simulink model "impedance_target"  (R2021b)
settings: Solver=ode1  StartTime=0.0  StopTime=inf  FixedStep=2e-4  RelTol=1e-3  EnableMultiTasking=on
InitFcn:
  | current_gain = 0.05;
libraries: spsSecondOrderFilterLib x4, speedgoatlib_IO102 x3, slrealtimeutilitieslib x1, slrealtimeiplib x1
settings Model: sg_rtwmakecfg_data=_sglibc_  SimulationMode=external  Creator=tcraddoc  LastModifiedBy=wasynczu
settings SolverCC: ConcurrentTasks=on  AlgebraicLoopSolver=TrustRegion  PositivePriorityOrder=on
settings DataIOCC: SaveFormat=StructureWithTime  ReturnWorkspaceOutputs=off
settings OptimizationCC: BlockReduction=off  OptimizeBlockIOStorage=off  BufferReuse=off  GlobalBufferReuse=off  ExpressionFolding=off  LocalBlockOutputs=off  OptimizeDataStoreBuffers=off  BusAssignmentInplaceUpdate=off
settings DebuggingCC: TasksWithSamePriorityMsg=none  SFMachineParentedDataDiag=warning  ArithmeticOperatorsInVariantConditions=warning
settings HardwareCC: ProdBitPerLong=64  ProdLongLongMode=on  ProdHWDeviceType=Intel->x86-64 (Linux 64)
settings SFSimCC: SimUseLocalCustomCode=off  CustomCodeUndefinedFunction=UseInterfaceOnly
settings RTWCC: Description=Simulink Real-Time  SystemTargetFile=slrealtime.tlc  TemplateMakefile=slrealtime_default_tmf  RTWUseLocalCustomCode=off  Toolchain=Simulink Real-Time Toolchain  BuildConfiguration=Faster Runs  CodeExecutionProfiling=on  TargetLang=C++
settings CodeAppCC: StateflowObjectComments=on
settings SimscapeCC: SimscapeNormalizeSystem=off

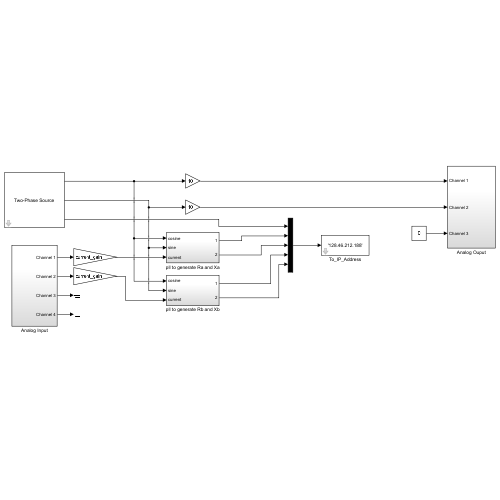
[thumbnail: Simulink's stored preview of the top-level diagram]
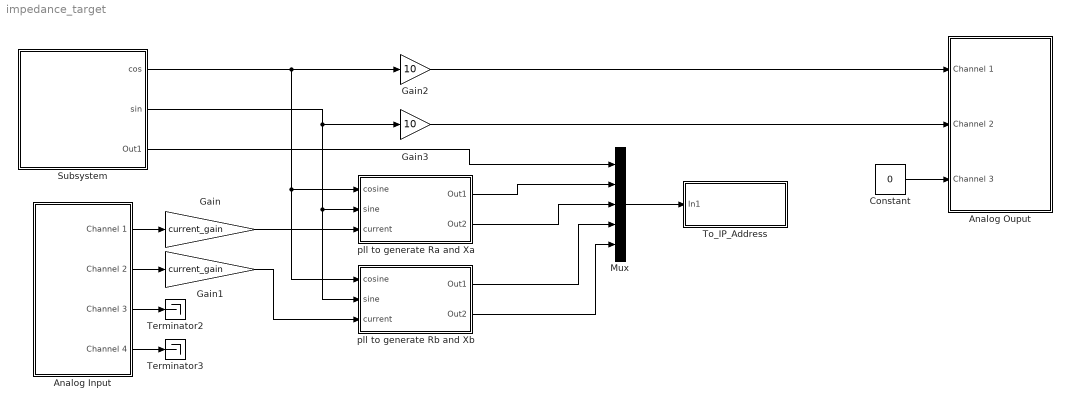
== system impedance_target ==
  Analog Input : Subsystem
  Analog Ouput : Subsystem
  Constant : Constant  Value=0
  Gain : Gain  Gain=current_gain
  Gain1 : Gain  Gain=current_gain
  Gain2 : Gain  Gain=10
  Gain3 : Gain  Gain=10
  Mux : Mux  Inputs=5
  Subsystem : Subsystem  mask{freq=10}
      mask prompts: freq "Frequency (Hz)"
      mask Display: disp('Two-Phase Source')
  Terminator2 : Terminator
  Terminator3 : Terminator
  To_IP_Address : Subsystem  mask{toAddress='128.46.212.188'}
      mask prompts: toAddress "To IP address"
      mask Display: disp(get_param(gcb,'toAddress'))
  pll to generate Ra and Xa : Subsystem
  pll to generate Rb and Xb : Subsystem
  wires:
  Subsystem/1(cos) -> pll to generate Rb and Xb/1(cosine), pll to generate Ra and Xa/1(cosine), Gain2/1
  Constant/1 -> Analog Ouput/3(Channel 3)
  Analog Input/1(Channel 1) -> Gain/1
  Analog Input/2(Channel 2) -> Gain1/1
  Analog Input/4(Channel 4) -> Terminator3/1
  Analog Input/3(Channel 3) -> Terminator2/1
  Subsystem/2(sin) -> pll to generate Rb and Xb/2(sine), pll to generate Ra and Xa/2(sine), Gain3/1
  Gain/1 -> pll to generate Ra and Xa/3(current)
  Gain1/1 -> pll to generate Rb and Xb/3(current)
  Gain2/1 -> Analog Ouput/1(Channel 1)
  Gain3/1 -> Analog Ouput/2(Channel 2)
  Subsystem/3(Out1) -> Mux/1
  pll to generate Ra and Xa/1(Out1) -> Mux/2
  pll to generate Ra and Xa/2(Out2) -> Mux/3
  pll to generate Rb and Xb/1(Out1) -> Mux/4
  pll to generate Rb and Xb/2(Out2) -> Mux/5
  Mux/1 -> To_IP_Address/1(In1)

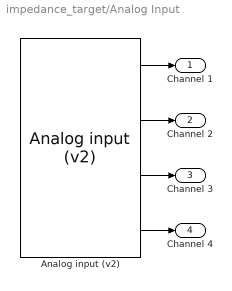
== system impedance_target/Analog Input ==
  "Analog input (v2) " : speedgoatlib_IO102/Analog input (v2)   id=1  channels=[1 2 3 4]  range=1  high_voltage=off  adCoupling=2  ts=2e-4  pciSlot=-1
      settings: SourceProductName=Simulink Real-Time: Speedgoat I/O Blockset
  Channel 1 : Outport
  Channel 2 : Outport  Port=2
  Channel 3 : Outport  Port=3
  Channel 4 : Outport  Port=4
  wires:
  "Analog input (v2) "/4 -> Channel 4/1
  "Analog input (v2) "/2 -> Channel 2/1
  "Analog input (v2) "/1 -> Channel 1/1
  "Analog input (v2) "/3 -> Channel 3/1

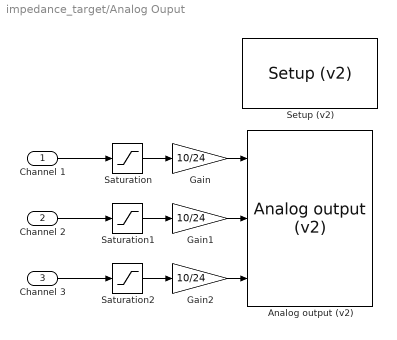
== system impedance_target/Analog Ouput ==
  Channel 1 : Inport
  Channel 2 : Inport  Port=2
  Channel 3 : Inport  Port=3
  "Analog output (v2) " : speedgoatlib_IO102/Analog output (v2)   id=1  channels=[1 2 3]  range=1  ts=2e-4  pciSlot=-1
      settings: SourceProductName=Simulink Real-Time: Speedgoat I/O Blockset
  Gain : Gain  Gain=10/24
  Gain1 : Gain  Gain=10/24
  Gain2 : Gain  Gain=10/24
  Saturation : Saturate  UpperLimit=24  LowerLimit=-24
  Saturation1 : Saturate  UpperLimit=24  LowerLimit=-24
  Saturation2 : Saturate  UpperLimit=24  LowerLimit=-24
  "Setup (v2) " : speedgoatlib_IO102/Setup (v2)   id=1  range=+-10V  cal=off  pciSlot=-1  adCoupling=Single-ended  adChannelMode=Multiple-channel (enter number of channels below)  adChannel=4  daChannel=[1,2,3]  daInitValue=[0]  daReset=[1]  DioDirectionLo=Input  DioDirectionHi=Output  doChannel=[9]  doInitValue=[0]  doReset=[1]  diChannel=[1]
      settings: SourceProductName=Simulink Real-Time: Speedgoat I/O Blockset
  wires:
  Saturation/1 -> Gain/1
  Saturation1/1 -> Gain1/1
  Saturation2/1 -> Gain2/1
  Gain1/1 -> "Analog output (v2) "/2
  Gain/1 -> "Analog output (v2) "/1
  Gain2/1 -> "Analog output (v2) "/3
  Channel 2/1 -> Saturation1/1
  Channel 3/1 -> Saturation2/1
  Channel 1/1 -> Saturation/1

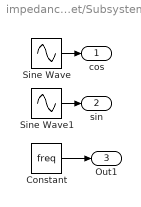
== system impedance_target/Subsystem ==
  Constant : Constant  Value=freq
  Sine Wave : Sin  Frequency=2*pi*freq  Phase=pi/2  SampleTime=0
  Sine Wave1 : Sin  Frequency=2*pi*freq  SampleTime=0
  cos : Outport  VectorParamsAs1DForOutWhenUnconnected=off
  sin : Outport  Port=2  VectorParamsAs1DForOutWhenUnconnected=off
  Out1 : Outport  Port=3
  wires:
  Sine Wave1/1 -> sin/1
  Sine Wave/1 -> cos/1
  Constant/1 -> Out1/1

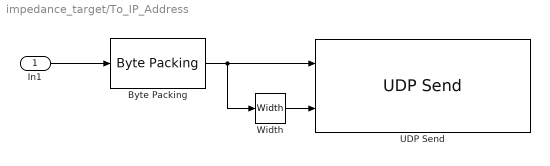
== system impedance_target/To_IP_Address ==
  In1 : Inport
  Byte Packing : slrealtimeutilitieslib/Byte Packing  MaskPackedDataType=uint8  MaskUnpackedDataTypes={['double']}  MaskAlignment=1
  UDP Send : slrealtimeiplib/UDP Send  useHostTargetConn=on  toAddress=toAddress  toPort=34  sampleTime=-1
      settings: SourceProductBaseCode=XP
  Width : Width
  wires:
  In1/1 -> Byte Packing/1
  Byte Packing/1 -> Width/1, UDP Send/1
  Width/1 -> UDP Send/2

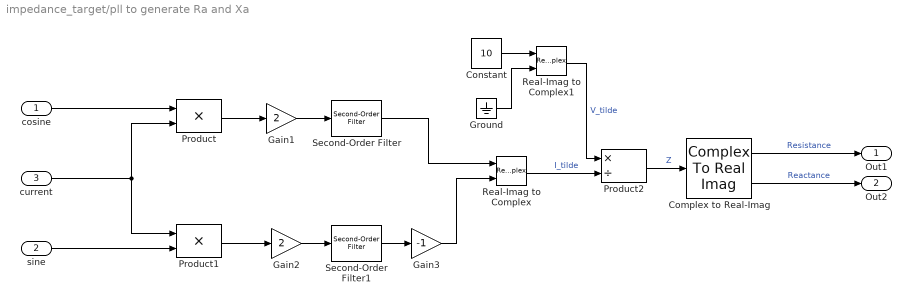
== system impedance_target/pll to generate Ra and Xa ==
  cosine : Inport
  sine : Inport  Port=2
  current : Inport  Port=3
  Complex to Real-Imag : ComplexToRealImag
  Constant : Constant  Value=10
  Gain1 : Gain  Gain=2  SaturateOnIntegerOverflow=on  OutDataTypeStr=Inherit: Same as input  ParamDataTypeStr=Inherit: Same as input
  Gain2 : Gain  Gain=2  SaturateOnIntegerOverflow=on  OutDataTypeStr=Inherit: Same as input  ParamDataTypeStr=Inherit: Same as input
  Gain3 : Gain  Gain=-1  SaturateOnIntegerOverflow=on  OutDataTypeStr=Inherit: Same as input  ParamDataTypeStr=Inherit: Same as input
  Ground : Ground
  Product : Product  InputSameDT=on  SaturateOnIntegerOverflow=on  OutDataTypeStr=Inherit: Same as first input
  Product1 : Product  InputSameDT=on  SaturateOnIntegerOverflow=on  OutDataTypeStr=Inherit: Same as first input
  Product2 : Product  Inputs=*/  InputSameDT=on  SaturateOnIntegerOverflow=on  OutDataTypeStr=Inherit: Same as first input
  Real-Imag to Complex : RealImagToComplex
  Real-Imag to Complex1 : RealImagToComplex
  Second-Order Filter : spsSecondOrderFilterLib/Second-Order Filter  FilterType=Lowpass  Fo=0.1  Zeta=0.707  Ts=0  Initialize=off  Vac_Init="[0,  0,  60]"  Vdc_Init=0  PlotResponse=off  FreqRange=[0, 500, 1]
      settings: SourceProductBaseCode=PS
  Second-Order Filter1 : spsSecondOrderFilterLib/Second-Order Filter  FilterType=Lowpass  Fo=0.1  Zeta=0.707  Ts=0  Initialize=off  Vac_Init="[0,  0,  60]"  Vdc_Init=0  PlotResponse=off  FreqRange=[0, 500, 1]
      settings: SourceProductBaseCode=PS
  Out1 : Outport
  Out2 : Outport  Port=2
  wires:
  Gain3/1 -> Real-Imag to Complex/2
  Complex to Real-Imag/2 -> Out2/1  "Reactance"
  Complex to Real-Imag/1 -> Out1/1  "Resistance"
  Product2/1 -> Complex to Real-Imag/1  "Z"
  Real-Imag to Complex1/1 -> Product2/1  "V_tilde"
  Ground/1 -> Real-Imag to Complex1/2
  Constant/1 -> Real-Imag to Complex1/1
  Real-Imag to Complex/1 -> Product2/2  "I_tilde"
  current/1 -> Product/2, Product1/1
  cosine/1 -> Product/1
  Gain1/1 -> Second-Order Filter/1
  Gain2/1 -> Second-Order Filter1/1
  Product1/1 -> Gain2/1
  Product/1 -> Gain1/1
  sine/1 -> Product1/2
  Second-Order Filter1/1 -> Gain3/1
  Second-Order Filter/1 -> Real-Imag to Complex/1

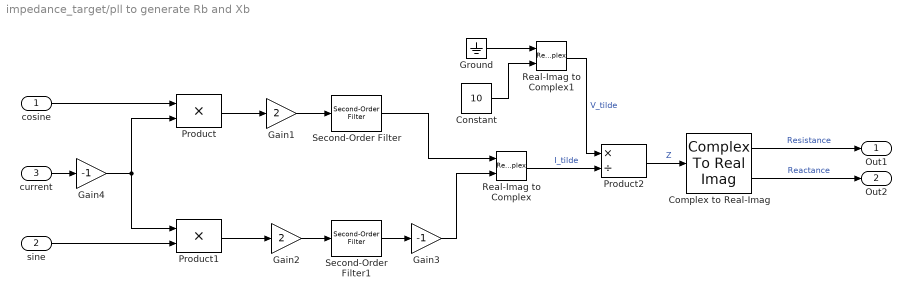
== system impedance_target/pll to generate Rb and Xb ==
  cosine : Inport
  sine : Inport  Port=2
  current : Inport  Port=3
  Complex to Real-Imag : ComplexToRealImag
  Constant : Constant  Value=10
  Gain1 : Gain  Gain=2  SaturateOnIntegerOverflow=on  OutDataTypeStr=Inherit: Same as input  ParamDataTypeStr=Inherit: Same as input
  Gain2 : Gain  Gain=2  SaturateOnIntegerOverflow=on  OutDataTypeStr=Inherit: Same as input  ParamDataTypeStr=Inherit: Same as input
  Gain3 : Gain  Gain=-1  SaturateOnIntegerOverflow=on  OutDataTypeStr=Inherit: Same as input  ParamDataTypeStr=Inherit: Same as input
  Gain4 : Gain  Gain=-1  SaturateOnIntegerOverflow=on  OutDataTypeStr=Inherit: Same as input  ParamDataTypeStr=Inherit: Same as input
  Ground : Ground
  Product : Product  InputSameDT=on  SaturateOnIntegerOverflow=on  OutDataTypeStr=Inherit: Same as first input
  Product1 : Product  InputSameDT=on  SaturateOnIntegerOverflow=on  OutDataTypeStr=Inherit: Same as first input
  Product2 : Product  Inputs=*/  InputSameDT=on  SaturateOnIntegerOverflow=on  OutDataTypeStr=Inherit: Same as first input
  Real-Imag to Complex : RealImagToComplex
  Real-Imag to Complex1 : RealImagToComplex
  Second-Order Filter : spsSecondOrderFilterLib/Second-Order Filter  FilterType=Lowpass  Fo=0.1  Zeta=0.707  Ts=0  Initialize=off  Vac_Init="[0,  0,  60]"  Vdc_Init=0  PlotResponse=off  FreqRange=[0, 500, 1]
      settings: SourceProductBaseCode=PS
  Second-Order Filter1 : spsSecondOrderFilterLib/Second-Order Filter  FilterType=Lowpass  Fo=0.1  Zeta=0.707  Ts=0  Initialize=off  Vac_Init="[0,  0,  60]"  Vdc_Init=0  PlotResponse=off  FreqRange=[0, 500, 1]
      settings: SourceProductBaseCode=PS
  Out1 : Outport
  Out2 : Outport  Port=2
  wires:
  Second-Order Filter/1 -> Real-Imag to Complex/1
  Second-Order Filter1/1 -> Gain3/1
  sine/1 -> Product1/2
  Product/1 -> Gain1/1
  Product1/1 -> Gain2/1
  Gain2/1 -> Second-Order Filter1/1
  Gain1/1 -> Second-Order Filter/1
  cosine/1 -> Product/1
  current/1 -> Gain4/1
  Real-Imag to Complex/1 -> Product2/2  "I_tilde"
  Real-Imag to Complex1/1 -> Product2/1  "V_tilde"
  Product2/1 -> Complex to Real-Imag/1  "Z"
  Complex to Real-Imag/1 -> Out1/1  "Resistance"
  Complex to Real-Imag/2 -> Out2/1  "Reactance"
  Gain3/1 -> Real-Imag to Complex/2
  Ground/1 -> Real-Imag to Complex1/1
  Constant/1 -> Real-Imag to Complex1/2
  Gain4/1 -> Product1/1, Product/2
